simulink model "Stationary "  (R2023b)
settings: Solver=VariableStepAuto  StartTime=0.0  StopTime=0.05  RelTol=1e-3
settings Model: Creator=Akaashdeep B  LastModifiedBy=Akaashdeep B

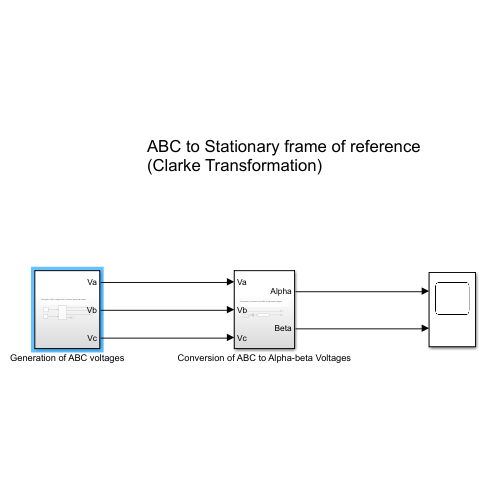
[thumbnail: Simulink's stored preview of the top-level diagram]
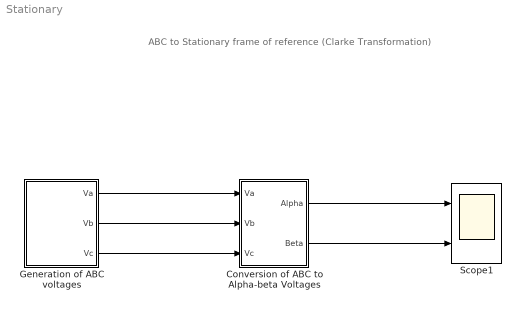
== system Stationary  ==
  note: ABC to Stationary frame of reference
      | (Clarke Transformation)
  Conversion of ABC to Alpha-beta Voltages : Subsystem
  Generation of ABC voltages : Subsystem
  Scope1 : Scope  NumInputPorts=2
  wires:
  Conversion of ABC to Alpha-beta Voltages/1(Alpha) -> Scope1/1
  Conversion of ABC to Alpha-beta Voltages/2(Beta) -> Scope1/2
  Generation of ABC voltages/1(Va) -> Conversion of ABC to Alpha-beta Voltages/1(Va)
  Generation of ABC voltages/2(Vb) -> Conversion of ABC to Alpha-beta Voltages/2(Vb)
  Generation of ABC voltages/3(Vc) -> Conversion of ABC to Alpha-beta Voltages/3(Vc)

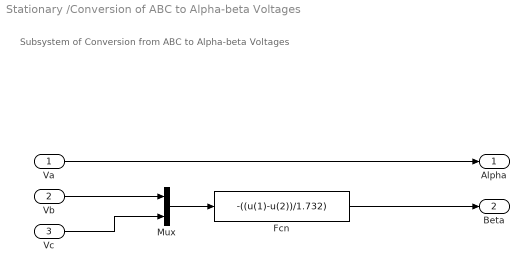
== system Stationary /Conversion of ABC to Alpha-beta Voltages ==
  note: Subsystem of Conversion from ABC to Alpha-beta Voltages
  Va : Inport
  Vb : Inport  Port=2
  Vc : Inport  Port=3
  Fcn : Fcn  Expr=-((u(1)-u(2))/1.732)
  Mux : Mux  Inputs=2
  Alpha : Outport
  Beta : Outport  Port=2
  wires:
  Mux/1 -> Fcn/1
  Fcn/1 -> Beta/1
  Vc/1 -> Mux/2
  Vb/1 -> Mux/1
  Va/1 -> Alpha/1

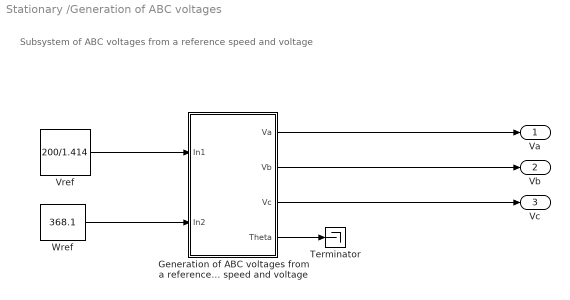
== system Stationary /Generation of ABC voltages ==
  note: Subsystem of ABC voltages from a reference speed and voltage
  "Generation of ABC voltages from a reference speed and voltage " : Subsystem
  Terminator : Terminator
  Vref : Constant  Value=200/1.414
  Wref : Constant  Value=368.1
  Va : Outport
  Vb : Outport  Port=2
  Vc : Outport  Port=3
  wires:
  Wref/1 -> "Generation of ABC voltages from a reference speed and voltage "/2(In2)
  Vref/1 -> "Generation of ABC voltages from a reference speed and voltage "/1(In1)
  "Generation of ABC voltages from a reference speed and voltage "/2(Vb) -> Vb/1
  "Generation of ABC voltages from a reference speed and voltage "/3(Vc) -> Vc/1
  "Generation of ABC voltages from a reference speed and voltage "/1(Va) -> Va/1
  "Generation of ABC voltages from a reference speed and voltage "/4(Theta) -> Terminator/1

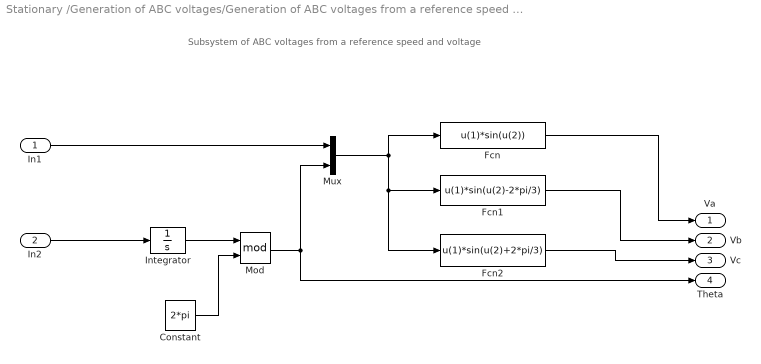
== system Stationary /Generation of ABC voltages/Generation of ABC voltages from a reference speed and voltage  ==
  note: Subsystem of ABC voltages from a reference speed and voltage
  In1 : Inport
  In2 : Inport  Port=2
  Constant : Constant  Value=2*pi
  Fcn : Fcn  Expr=u(1)*sin(u(2))
  Fcn1 : Fcn  Expr=u(1)*sin(u(2)-2*pi/3)
  Fcn2 : Fcn  Expr=u(1)*sin(u(2)+2*pi/3)
  Integrator : Integrator
  Mod : Math  Operator=mod
  Mux : Mux  Inputs=2
  Va : Outport
  Vb : Outport  Port=2
  Vc : Outport  Port=3
  Theta : Outport  Port=4
  wires:
  Mod/1 -> Theta/1, Mux/2
  Constant/1 -> Mod/2
  Mux/1 -> Fcn2/1, Fcn1/1, Fcn/1
  Fcn1/1 -> Vb/1
  Integrator/1 -> Mod/1
  Fcn/1 -> Va/1
  In1/1 -> Mux/1
  Fcn2/1 -> Vc/1
  In2/1 -> Integrator/1
